simulink model "uas_main_latest"  (R2025a)
settings: Solver=FixedStepAuto  StartTime=0.0  StopTime=Inf  FixedStep=sample_time  RelTol=1e-3
model workspace: external: MAT-File (data not in the file)
values from neighbouring files (symbols this model uses):
  arm_length = 0.17    [test_uas_parameters.m]    (also in uas_parameters.m; uas_parameters_akin.m; uas_parameters_brushless.m = 0.046)
  drag_coefficient = 0.47    [uas_parameters.m]    (also in uas_parameters_akin.m; uas_parameters_brushless.m)
  g = 9.80665    [test_uas_parameters.m]    (also in uas_parameters.m; uas_parameters_akin.m; uas_parameters_brushless.m)
  inertia_xx = 0.007    [test_uas_parameters.m]    (also in uas_parameters.m; uas_parameters_akin.m; uas_parameters_brushless.m = 1.657171e-05)
  inertia_yy = 0.007    [test_uas_parameters.m]    (also in uas_parameters.m; uas_parameters_akin.m; uas_parameters_brushless.m = 1.6655602e-05)
  inertia_zz = 0.012    [test_uas_parameters.m]    (also in uas_parameters.m; uas_parameters_akin.m; uas_parameters_brushless.m = 2.9261652e-05)
  mass_drone = 0.68    [test_uas_parameters.m]    (also in uas_parameters.m; uas_parameters_akin.m; uas_parameters_brushless.m = 0.037)
  mass_total = mass_drone    (= 0.68)    [test_uas_parameters.m]    (also in uas_parameters.m; uas_parameters_akin.m; uas_parameters_brushless.m = 0.037)
  max_rot_velocity = 838    [uas_parameters.m]    (also in uas_parameters_akin.m; uas_parameters_brushless.m)
  mix_matrix = inv(motor_constant * allocation_matrix)    [test_uas_parameters.m]    (also in uas_parameters.m; uas_parameters_akin.m; uas_parameters_brushless.m)
  moment_constant = 0.016    [test_uas_parameters.m]    (also in uas_parameters.m; uas_parameters_akin.m; uas_parameters_brushless.m = 0.006)
  motor_constant = 8.54858e-06    [test_uas_parameters.m]    (also in uas_parameters.m; uas_parameters_akin.m; uas_parameters_brushless.m = 1.45e-08)
  publish_rate = sample_time    (= 0.04)    [test_uas_parameters.m]    (also in uas_parameters.m; uas_parameters_akin.m; uas_parameters_brushless.m)
  reference_area = pi * (75e-3)^2    (= 0.0176714586764)    [uas_parameters.m]    (also in uas_parameters_akin.m; uas_parameters_brushless.m)
  rotor_offset_top = 0.01    [uas_parameters.m]    (also in uas_parameters_akin.m; uas_parameters_brushless.m)
  route = route_scaled    [generate_route_for_simulink.m]    (also in uas_parameters.m = route_smooth; uas_parameters_akin.m = route_dense; uas_parameters_brushless.m = [0 0 1 ; 9 0 1 ; 9 9 1])
  sample_time = 4e-2    (= 0.04)    [test_uas_parameters.m]    (also in uas_parameters.m; uas_parameters_akin.m; uas_parameters_brushless.m)
  x0 = route_world(1,1)    [uas_parameters.m]    (also in uas_parameters_akin.m = route(1,1); uas_parameters_brushless.m = 36)
  y0 = route_world(1,2)    [uas_parameters.m]    (also in uas_parameters_akin.m = route(1,2); uas_parameters_brushless.m = 80)
  z0 = route_world(1,3)    [uas_parameters.m]    (also in uas_parameters_akin.m = route(1,3); uas_parameters_brushless.m = 1)
undefined symbols (not defined in the file or in its folder): Angular, Linear, poly_traj, Position, quat2rotm, X, Y, Z
libraries: nesl_utility x32, sm_lib x25, ros2lib x8, sim3dlib x1, uavsim3dlib x1, simulink x1, vrlib x1, simulink_extras x1
(part 2 of 2)

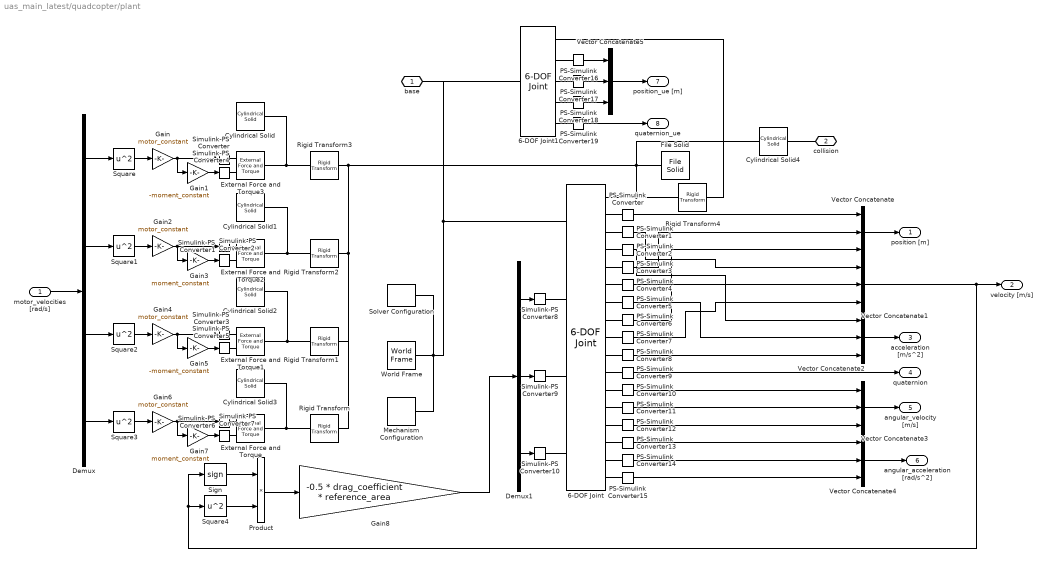
== system uas_main_latest/quadcopter/plant ==
  motor_velocities [rad/s] : Inport
  6-DOF Joint : sm_lib/Joints/6-DOF Joint  JointMode=Normal  CompositeWrenchDir=BaseOnFollower  CompositeWrenchFrame=BaseFrame  SenseConstraintForce=off  SenseConstraintTorque=off  SenseTotalForce=off  SenseTotalTorque=off  PxPositionTargetSpecify=on  PxPositionTargetPriority=High  PxPositionTargetValue=0  PxPositionTargetValueUnits=m  PxVelocityTargetSpecify=off  PxVelocityTargetPriority=High  PxVelocityTargetValue=0  PxVelocityTargetValueUnits=m/s  PxEquilibriumPosition=0  PxEquilibriumPositionUnits=m  PxSpringStiffness=0  PxSpringStiffnessUnits=N/m  PxDampingCoefficient=0  PxDampingCoefficientUnits=N/(m/s)  PxLowerLimitSpecify=off  PxLowerLimitBound=-1  PxLowerLimitBoundUnits=m  PxLowerLimitStiffness=1e6  PxLowerLimitStiffnessUnits=N/m  PxLowerLimitDamping=1e3  PxLowerLimitDampingUnits=N/(m/s)  PxLowerLimitTransitionRegionWidth=1e-4  PxLowerLimitTransitionRegionWidthUnits=m  PxUpperLimitSpecify=off  PxUpperLimitBound=1  PxUpperLimitBoundUnits=m  PxUpperLimitStiffness=1e6  PxUpperLimitStiffnessUnits=N/m  PxUpperLimitDamping=1e3  PxUpperLimitDampingUnits=N/(m/s)  PxUpperLimitTransitionRegionWidth=1e-4  PxUpperLimitTransitionRegionWidthUnits=m  PxTorqueActuationMode=InputTorque  PxMotionActuationMode=ComputedMotion  PxSensePosition=on  PxSenseVelocity=on  PxSenseAcceleration=on  PxSenseTorqueForce=off  PxSenseLowerLimitTorqueForce=off  PxSenseUpperLimitTorqueForce=off  PyPositionTargetSpecify=on  PyPositionTargetPriority=High  PyPositionTargetValue=0  PyPositionTargetValueUnits=m  PyVelocityTargetSpecify=off  PyVelocityTargetPriority=High  PyVelocityTargetValue=0  PyVelocityTargetValueUnits=m/s  PyEquilibriumPosition=0  PyEquilibriumPositionUnits=m  PySpringStiffness=0  PySpringStiffnessUnits=N/m  PyDampingCoefficient=0  PyDampingCoefficientUnits=N/(m/s)  PyLowerLimitSpecify=off  PyLowerLimitBound=-1  PyLowerLimitBoundUnits=m  PyLowerLimitStiffness=1e6  PyLowerLimitStiffnessUnits=N/m  PyLowerLimitDamping=1e3  PyLowerLimitDampingUnits=N/(m/s)  PyLowerLimitTransitionRegionWidth=1e-4  PyLowerLimitTransitionRegionWidthUnits=m  PyUpperLimitSpecify=off  PyUpperLimitBound=1  PyUpperLimitBoundUnits=m  PyUpperLimitStiffness=1e6  PyUpperLimitStiffnessUnits=N/m  PyUpperLimitDamping=1e3  PyUpperLimitDampingUnits=N/(m/s)  PyUpperLimitTransitionRegionWidth=1e-4  PyUpperLimitTransitionRegionWidthUnits=m  PyTorqueActuationMode=InputTorque  PyMotionActuationMode=ComputedMotion  PySensePosition=on  PySenseVelocity=on  PySenseAcceleration=on  PySenseTorqueForce=off  PySenseLowerLimitTorqueForce=off  PySenseUpperLimitTorqueForce=off  PzPositionTargetSpecify=on  PzPositionTargetPriority=High  PzPositionTargetValue=z0  PzPositionTargetValueUnits=m  PzVelocityTargetSpecify=off  PzVelocityTargetPriority=High  PzVelocityTargetValue=0  PzVelocityTargetValueUnits=m/s  PzEquilibriumPosition=0  PzEquilibriumPositionUnits=m  PzSpringStiffness=0  PzSpringStiffnessUnits=N/m  PzDampingCoefficient=0  PzDampingCoefficientUnits=N/(m/s)  PzLowerLimitSpecify=off  PzLowerLimitBound=-1  PzLowerLimitBoundUnits=m  PzLowerLimitStiffness=1e6  PzLowerLimitStiffnessUnits=N/m  PzLowerLimitDamping=1e3  PzLowerLimitDampingUnits=N/(m/s)  PzLowerLimitTransitionRegionWidth=1e-4  PzLowerLimitTransitionRegionWidthUnits=m  PzUpperLimitSpecify=off  PzUpperLimitBound=1  PzUpperLimitBoundUnits=m  PzUpperLimitStiffness=1e6  PzUpperLimitStiffnessUnits=N/m  PzUpperLimitDamping=1e3  PzUpperLimitDampingUnits=N/(m/s)  PzUpperLimitTransitionRegionWidth=1e-4  PzUpperLimitTransitionRegionWidthUnits=m  PzTorqueActuationMode=InputTorque  PzMotionActuationMode=ComputedMotion  PzSensePosition=on  PzSenseVelocity=on  PzSenseAcceleration=on  PzSenseTorqueForce=off  PzSenseLowerLimitTorqueForce=off  PzSenseUpperLimitTorqueForce=off  SphPositionTargetSpecify=on  SphPositionTargetPriority=High  SphPositionTargetRotationMethod=StandardAxis  SphPositionTargetFollAlignAxisA=+X  SphPositionTargetBaseAlignAxisA=+Y  SphPositionTargetFollAlignAxisB=+Y  SphPositionTargetBaseAlignAxisB=+Z  SphPositionTargetRotationStandardAxis=+Z  SphPositionTargetRotationAngle=0  SphPositionTargetRotationAngleUnits=deg  SphPositionTargetRotationArbitraryAxis=[0 0 1]  SphPositionTargetRotationSequenceAxes=FollowerAxes  SphPositionTargetRotationSequence=XYX  SphPositionTargetRotationSequenceAngles=[0 0 0]  SphPositionTargetRotationSequenceAnglesUnits=deg  SphPositionTargetRotationMatrix=[1 0 0; 0 1 0; 0 0 1]  SphPositionTargetQuaternion=[1 0 0 0]  SphVelocityTargetSpecify=off  SphVelocityTargetPriority=High  SphVelocityTargetValue=[0 0 0]  SphVelocityTargetValueUnits=deg/s  SphVelocityTargetInFollowerFrame=on  SphEqPosRotationMethod=None  SphEqPosFollAlignAxisA=+X  SphEqPosBaseAlignAxisA=+Y  SphEqPosFollAlignAxisB=+Y  SphEqPosBaseAlignAxisB=+Z  SphEqPosRotationStandardAxis=+Z  SphEqPosRotationAngle=0.0  SphEqPosRotationAngleUnits=deg  SphEqPosRotationArbitraryAxis=[0 0 1]  SphEqPosRotationSequenceAxes=FollowerAxes  SphEqPosRotationSequence=XYX  SphEqPosRotationSequenceAngles=[0 0 0]  SphEqPosRotationSequenceAnglesUnits=deg  SphEqPosRotationMatrix=[1 0 0; 0 1 0; 0 0 1]  SphEqPosQuaternion=[1 0 0 0]  SphSpringStiffness=0  SphSpringStiffnessUnits=N*m/deg  SphDampingCoefficient=0  SphDampingCoefficientUnits=N*m/(deg/s)  SphLowerLimitSpecify=off  SphLowerLimitBound=15  SphLowerLimitBoundUnits=deg  SphLowerLimitStiffness=1e4  SphLowerLimitStiffnessUnits=N*m/deg  SphLowerLimitDamping=10  SphLowerLimitDampingUnits=N*m/(deg/s)  SphLowerLimitTransitionRegionWidth=0.1  SphLowerLimitTransitionRegionWidthUnits=deg  SphUpperLimitSpecify=off  SphUpperLimitBound=45  SphUpperLimitBoundUnits=deg  SphUpperLimitStiffness=1e4  SphUpperLimitStiffnessUnits=N*m/deg  SphUpperLimitDamping=10  SphUpperLimitDampingUnits=N*m/(deg/s)  SphUpperLimitTransitionRegionWidth=0.1  SphUpperLimitTransitionRegionWidthUnits=deg  SphTorqueActuationMode=NoTorque  SphActuateTorqueX=off  SphActuateTorqueY=off  SphActuateTorqueZ=off  SphActuateTorque=off  SphActuationFrame=BaseFrame  SphSensePosition=on  SphSenseVelocityX=on  SphSenseVelocityY=on  SphSenseVelocityZ=on  SphSenseVelocity=off  SphSenseAccelerationX=on  SphSenseAccelerationY=on  SphSenseAccelerationZ=on  SphSenseAcceleration=off  SphSenseLowerLimitTorqueMag=off  SphSenseUpperLimitTorqueMag=off  SphSensingFrame=BaseFrame
  6-DOF Joint1 : sm_lib/Joints/6-DOF Joint  JointMode=Normal  CompositeWrenchDir=FollowerOnBase  CompositeWrenchFrame=BaseFrame  SenseConstraintForce=off  SenseConstraintTorque=off  SenseTotalForce=off  SenseTotalTorque=off  PxPositionTargetSpecify=off  PxPositionTargetPriority=High  PxPositionTargetValue=0  PxPositionTargetValueUnits=m  PxVelocityTargetSpecify=off  PxVelocityTargetPriority=High  PxVelocityTargetValue=0  PxVelocityTargetValueUnits=m/s  PxEquilibriumPosition=0  PxEquilibriumPositionUnits=m  PxSpringStiffness=0  PxSpringStiffnessUnits=N/m  PxDampingCoefficient=0  PxDampingCoefficientUnits=N/(m/s)  PxLowerLimitSpecify=off  PxLowerLimitBound=-1  PxLowerLimitBoundUnits=m  PxLowerLimitStiffness=1e6  PxLowerLimitStiffnessUnits=N/m  PxLowerLimitDamping=1e3  PxLowerLimitDampingUnits=N/(m/s)  PxLowerLimitTransitionRegionWidth=1e-4  PxLowerLimitTransitionRegionWidthUnits=m  PxUpperLimitSpecify=off  PxUpperLimitBound=1  PxUpperLimitBoundUnits=m  PxUpperLimitStiffness=1e6  PxUpperLimitStiffnessUnits=N/m  PxUpperLimitDamping=1e3  PxUpperLimitDampingUnits=N/(m/s)  PxUpperLimitTransitionRegionWidth=1e-4  PxUpperLimitTransitionRegionWidthUnits=m  PxTorqueActuationMode=NoTorque  PxMotionActuationMode=ComputedMotion  PxSensePosition=on  PxSenseVelocity=off  PxSenseAcceleration=off  PxSenseTorqueForce=off  PxSenseLowerLimitTorqueForce=off  PxSenseUpperLimitTorqueForce=off  PyPositionTargetSpecify=off  PyPositionTargetPriority=High  PyPositionTargetValue=0  PyPositionTargetValueUnits=m  PyVelocityTargetSpecify=off  PyVelocityTargetPriority=High  PyVelocityTargetValue=0  PyVelocityTargetValueUnits=m/s  PyEquilibriumPosition=0  PyEquilibriumPositionUnits=m  PySpringStiffness=0  PySpringStiffnessUnits=N/m  PyDampingCoefficient=0  PyDampingCoefficientUnits=N/(m/s)  PyLowerLimitSpecify=off  PyLowerLimitBound=-1  PyLowerLimitBoundUnits=m  PyLowerLimitStiffness=1e6  PyLowerLimitStiffnessUnits=N/m  PyLowerLimitDamping=1e3  PyLowerLimitDampingUnits=N/(m/s)  PyLowerLimitTransitionRegionWidth=1e-4  PyLowerLimitTransitionRegionWidthUnits=m  PyUpperLimitSpecify=off  PyUpperLimitBound=1  PyUpperLimitBoundUnits=m  PyUpperLimitStiffness=1e6  PyUpperLimitStiffnessUnits=N/m  PyUpperLimitDamping=1e3  PyUpperLimitDampingUnits=N/(m/s)  PyUpperLimitTransitionRegionWidth=1e-4  PyUpperLimitTransitionRegionWidthUnits=m  PyTorqueActuationMode=NoTorque  PyMotionActuationMode=ComputedMotion  PySensePosition=on  PySenseVelocity=off  PySenseAcceleration=off  PySenseTorqueForce=off  PySenseLowerLimitTorqueForce=off  PySenseUpperLimitTorqueForce=off  PzPositionTargetSpecify=off  PzPositionTargetPriority=High  PzPositionTargetValue=0  PzPositionTargetValueUnits=m  PzVelocityTargetSpecify=off  PzVelocityTargetPriority=High  PzVelocityTargetValue=0  PzVelocityTargetValueUnits=m/s  PzEquilibriumPosition=0  PzEquilibriumPositionUnits=m  PzSpringStiffness=0  PzSpringStiffnessUnits=N/m  PzDampingCoefficient=0  PzDampingCoefficientUnits=N/(m/s)  PzLowerLimitSpecify=off  PzLowerLimitBound=-1  PzLowerLimitBoundUnits=m  PzLowerLimitStiffness=1e6  PzLowerLimitStiffnessUnits=N/m  PzLowerLimitDamping=1e3  PzLowerLimitDampingUnits=N/(m/s)  PzLowerLimitTransitionRegionWidth=1e-4  PzLowerLimitTransitionRegionWidthUnits=m  PzUpperLimitSpecify=off  PzUpperLimitBound=1  PzUpperLimitBoundUnits=m  PzUpperLimitStiffness=1e6  PzUpperLimitStiffnessUnits=N/m  PzUpperLimitDamping=1e3  PzUpperLimitDampingUnits=N/(m/s)  PzUpperLimitTransitionRegionWidth=1e-4  PzUpperLimitTransitionRegionWidthUnits=m  PzTorqueActuationMode=NoTorque  PzMotionActuationMode=ComputedMotion  PzSensePosition=on  PzSenseVelocity=off  PzSenseAcceleration=off  PzSenseTorqueForce=off  PzSenseLowerLimitTorqueForce=off  PzSenseUpperLimitTorqueForce=off  SphPositionTargetSpecify=off  SphPositionTargetPriority=High  SphPositionTargetRotationMethod=None  SphPositionTargetFollAlignAxisA=+X  SphPositionTargetBaseAlignAxisA=+Y  SphPositionTargetFollAlignAxisB=+Y  SphPositionTargetBaseAlignAxisB=+Z  SphPositionTargetRotationStandardAxis=+Z  SphPositionTargetRotationAngle=0.0  SphPositionTargetRotationAngleUnits=deg  SphPositionTargetRotationArbitraryAxis=[0 0 1]  SphPositionTargetRotationSequenceAxes=FollowerAxes  SphPositionTargetRotationSequence=XYX  SphPositionTargetRotationSequenceAngles=[0 0 0]  SphPositionTargetRotationSequenceAnglesUnits=deg  SphPositionTargetRotationMatrix=[1 0 0; 0 1 0; 0 0 1]  SphPositionTargetQuaternion=[1 0 0 0]  SphVelocityTargetSpecify=off  SphVelocityTargetPriority=High  SphVelocityTargetValue=[0 0 0]  SphVelocityTargetValueUnits=deg/s  SphVelocityTargetInFollowerFrame=on  SphEqPosRotationMethod=None  SphEqPosFollAlignAxisA=+X  SphEqPosBaseAlignAxisA=+Y  SphEqPosFollAlignAxisB=+Y  SphEqPosBaseAlignAxisB=+Z  SphEqPosRotationStandardAxis=+Z  SphEqPosRotationAngle=0.0  SphEqPosRotationAngleUnits=deg  SphEqPosRotationArbitraryAxis=[0 0 1]  SphEqPosRotationSequenceAxes=FollowerAxes  SphEqPosRotationSequence=XYX  SphEqPosRotationSequenceAngles=[0 0 0]  SphEqPosRotationSequenceAnglesUnits=deg  SphEqPosRotationMatrix=[1 0 0; 0 1 0; 0 0 1]  SphEqPosQuaternion=[1 0 0 0]  SphSpringStiffness=0  SphSpringStiffnessUnits=N*m/deg  SphDampingCoefficient=0  SphDampingCoefficientUnits=N*m/(deg/s)  SphLowerLimitSpecify=off  SphLowerLimitBound=15  SphLowerLimitBoundUnits=deg  SphLowerLimitStiffness=1e4  SphLowerLimitStiffnessUnits=N*m/deg  SphLowerLimitDamping=10  SphLowerLimitDampingUnits=N*m/(deg/s)  SphLowerLimitTransitionRegionWidth=0.1  SphLowerLimitTransitionRegionWidthUnits=deg  SphUpperLimitSpecify=off  SphUpperLimitBound=45  SphUpperLimitBoundUnits=deg  SphUpperLimitStiffness=1e4  SphUpperLimitStiffnessUnits=N*m/deg  SphUpperLimitDamping=10  SphUpperLimitDampingUnits=N*m/(deg/s)  SphUpperLimitTransitionRegionWidth=0.1  SphUpperLimitTransitionRegionWidthUnits=deg  SphTorqueActuationMode=NoTorque  SphActuateTorqueX=off  SphActuateTorqueY=off  SphActuateTorqueZ=off  SphActuateTorque=off  SphActuationFrame=BaseFrame  SphSensePosition=on  SphSenseVelocityX=off  SphSenseVelocityY=off  SphSenseVelocityZ=off  SphSenseVelocity=off  SphSenseAccelerationX=off  SphSenseAccelerationY=off  SphSenseAccelerationZ=off  SphSenseAcceleration=off  SphSenseLowerLimitTorqueMag=off  SphSenseUpperLimitTorqueMag=off  SphSensingFrame=BaseFrame
  Cylindrical Solid : sm_lib/Body Elements/Cylindrical Solid  CylinderRadius=100  CylinderRadiusUnits=mm  CylinderLength=1  CylinderLengthUnits=mm  ExportEntireGeometry=off  InertiaType=CalculateFromGeometry  BasedOnType=Density  Density=0  DensityUnits=kg/m^3  Mass=1  MassUnits=kg  CenterOfMass=[0 0 0]  CenterOfMassUnits=m  MomentsOfInertia=[1 1 1]  MomentsOfInertiaUnits=kg*m^2  ProductsOfInertia=[0 0 0]  ProductsOfInertiaUnits=kg*m^2  GraphicType=FromGeometry  MarkerShape=Sphere  MarkerSize=10  GraphicVisPropType=SimpleVisualProperties  GraphicDiffuseColor=[1.0 0.0 0.0]  GraphicOpacity=0.5  GraphicSpecularColor=[0.5 0.5 0.5 1.0]  GraphicAmbientColor=[0.15 0.15 0.15 1.0]  GraphicEmissiveColor=[0.0 0.0 0.0 1.0]  GraphicShininess=75  DoExposeReferenceFrame=on  SerializedFrames=<Frames/>
  Cylindrical Solid1 : sm_lib/Body Elements/Cylindrical Solid  CylinderRadius=100  CylinderRadiusUnits=mm  CylinderLength=1  CylinderLengthUnits=mm  ExportEntireGeometry=off  InertiaType=CalculateFromGeometry  BasedOnType=Density  Density=0  DensityUnits=kg/m^3  Mass=1  MassUnits=kg  CenterOfMass=[0 0 0]  CenterOfMassUnits=m  MomentsOfInertia=[1 1 1]  MomentsOfInertiaUnits=kg*m^2  ProductsOfInertia=[0 0 0]  ProductsOfInertiaUnits=kg*m^2  GraphicType=FromGeometry  MarkerShape=Sphere  MarkerSize=10  GraphicVisPropType=SimpleVisualProperties  GraphicDiffuseColor=[0 1 0]  GraphicOpacity=0.5  GraphicSpecularColor=[0.5 0.5 0.5 1.0]  GraphicAmbientColor=[0.15 0.15 0.15 1.0]  GraphicEmissiveColor=[0.0 0.0 0.0 1.0]  GraphicShininess=75  DoExposeReferenceFrame=on  SerializedFrames=<Frames/>
  Cylindrical Solid2 : sm_lib/Body Elements/Cylindrical Solid  CylinderRadius=100  CylinderRadiusUnits=mm  CylinderLength=1  CylinderLengthUnits=mm  ExportEntireGeometry=off  InertiaType=CalculateFromGeometry  BasedOnType=Density  Density=0  DensityUnits=kg/m^3  Mass=1  MassUnits=kg  CenterOfMass=[0 0 0]  CenterOfMassUnits=m  MomentsOfInertia=[1 1 1]  MomentsOfInertiaUnits=kg*m^2  ProductsOfInertia=[0 0 0]  ProductsOfInertiaUnits=kg*m^2  GraphicType=FromGeometry  MarkerShape=Sphere  MarkerSize=10  GraphicVisPropType=SimpleVisualProperties  GraphicDiffuseColor=[0 0 1]  GraphicOpacity=0.5  GraphicSpecularColor=[0.5 0.5 0.5 1.0]  GraphicAmbientColor=[0.15 0.15 0.15 1.0]  GraphicEmissiveColor=[0.0 0.0 0.0 1.0]  GraphicShininess=75  DoExposeReferenceFrame=on  SerializedFrames=<Frames/>
  Cylindrical Solid3 : sm_lib/Body Elements/Cylindrical Solid  CylinderRadius=100  CylinderRadiusUnits=mm  CylinderLength=1  CylinderLengthUnits=mm  ExportEntireGeometry=off  InertiaType=CalculateFromGeometry  BasedOnType=Density  Density=0  DensityUnits=kg/m^3  Mass=1  MassUnits=kg  CenterOfMass=[0 0 0]  CenterOfMassUnits=m  MomentsOfInertia=[1 1 1]  MomentsOfInertiaUnits=kg*m^2  ProductsOfInertia=[0 0 0]  ProductsOfInertiaUnits=kg*m^2  GraphicType=FromGeometry  MarkerShape=Sphere  MarkerSize=10  GraphicVisPropType=SimpleVisualProperties  GraphicDiffuseColor=[0 0 1]  GraphicOpacity=0.5  GraphicSpecularColor=[0.5 0.5 0.5 1.0]  GraphicAmbientColor=[0.15 0.15 0.15 1.0]  GraphicEmissiveColor=[0.0 0.0 0.0 1.0]  GraphicShininess=75  DoExposeReferenceFrame=on  SerializedFrames=<Frames/>
  Cylindrical Solid4 : sm_lib/Body Elements/Cylindrical Solid  CylinderRadius=0.27  CylinderRadiusUnits=m  CylinderLength=0.3  CylinderLengthUnits=m  ExportEntireGeometry=on  InertiaType=CalculateFromGeometry  BasedOnType=Density  Density=0  DensityUnits=kg/m^3  Mass=1  MassUnits=kg  CenterOfMass=[0 0 0]  CenterOfMassUnits=m  MomentsOfInertia=[1 1 1]  MomentsOfInertiaUnits=kg*m^2  ProductsOfInertia=[0 0 0]  ProductsOfInertiaUnits=kg*m^2  GraphicType=FromGeometry  MarkerShape=Sphere  MarkerSize=10  GraphicVisPropType=SimpleVisualProperties  GraphicDiffuseColor=[0.5 0.5 0.5]  GraphicOpacity=0.2  GraphicSpecularColor=[0.5 0.5 0.5 1.0]  GraphicAmbientColor=[0.15 0.15 0.15 1.0]  GraphicEmissiveColor=[0.0 0.0 0.0 1.0]  GraphicShininess=75  DoExposeReferenceFrame=on  SerializedFrames=<Frames/>
  Demux : Demux
  Demux1 : Demux  Outputs=3
  External Force and Torque{,1..3} (4 alike) : sm_lib/Forces and Torques/External Force and Torque  EnableForceX=off  EnableForceY=off  EnableForceZ=on  EnableForce=off  ForceResolutionFrame=AttachedFrame  EnableTorqueX=off  EnableTorqueY=off  EnableTorqueZ=on  EnableTorque=off  TorqueResolutionFrame=AttachedFrame
  File Solid : sm_lib/Body Elements/File Solid  ExtGeomFileName=uas_geometry.stl  UnitType=Custom  ExtGeomFileUnits=m  StepReaderType=HEX  ExportConvexHullGeometry=off  InertiaType=Custom  BasedOnType=DensityFromFile  Density=1000  DensityUnits=kg/m^3  Mass=mass_drone  MassUnits=kg  CenterOfMass=[0 0 0]  CenterOfMassUnits=m  MomentsOfInertia=[inertia_xx inertia_yy inertia_zz]  MomentsOfInertiaUnits=kg*m^2  ProductsOfInertia=[0 0 0]  ProductsOfInertiaUnits=kg*m^2  GraphicType=FromGeometry  MarkerShape=Sphere  MarkerSize=10  GraphicVisPropType=SimpleVisualProperties  GraphicDiffuseColor=[1.0 1.0 1.0]  GraphicOpacity=1.0  GraphicSpecularColor=[0.5 0.5 0.5 1.0]  GraphicAmbientColor=[0.15 0.15 0.15 1.0]  GraphicEmissiveColor=[0.0 0.0 0.0 1.0]  GraphicShininess=75  DoExposeReferenceFrame=on  SerializedFrames=<Frames/>
  Gain{,2,4,6} (4 alike) : Gain  Gain=motor_constant
  Gain1 : Gain  Gain=-moment_constant
  Gain3 : Gain  Gain=moment_constant
  Gain5 : Gain  Gain=-moment_constant
  Gain7 : Gain  Gain=moment_constant
  Gain8 : Gain  Gain=-0.5 * drag_coefficient * reference_area
  Mechanism Configuration : sm_lib/Utilities/Mechanism Configuration  UniformGravity=Constant  GravityVector=[0 0 -9.80665]  GravityVectorUnits=m/s^2  LinearizationDelta=0.001  JointModeTransitionNonlinearIterations=2
  PS-Simulink Converter{,1..19} (20 alike) : nesl_utility/PS-Simulink Converter  PhysicalDomain=network_engine_domain  SubClassName=ps_output  LeftPortType=input  RightPortType=output  PseudoPeriodic=off  Frequencies=[]  VectorFormat=1-D array  Unit=inherit  AffineConversion=off
  Product : Product
  Rigid Transform : sm_lib/Frames and Transforms/Rigid Transform  RotationMethod=None  FollAlignAxisA=+X  BaseAlignAxisA=+Y  FollAlignAxisB=+Y  BaseAlignAxisB=+Z  RotationStandardAxis=+Z  RotationAngle=0.0  RotationAngleUnits=deg  RotationArbitraryAxis=[0 0 1]  RotationSequenceAxes=FollowerAxes  RotationSequence=XYX  RotationSequenceAngles=[0 0 0]  RotationSequenceAnglesUnits=deg  RotationMatrix=[1 0 0; 0 1 0; 0 0 1]  Quaternion=[1 0 0 0]  TranslationMethod=Cartesian  TranslationCartesianOffset=[0 -arm_length rotor_offset_top]  TranslationCartesianOffsetUnits=m  TranslationStandardAxis=+Z  TranslationStandardOffset=0  TranslationStandardOffsetUnits=m  TranslationROffset=0  TranslationROffsetUnits=m  TranslationThetaOffset=0  TranslationThetaOffsetUnits=deg  TranslationZOffset=0  TranslationZOffsetUnits=m
  Rigid Transform1 : sm_lib/Frames and Transforms/Rigid Transform  RotationMethod=None  FollAlignAxisA=+X  BaseAlignAxisA=+Y  FollAlignAxisB=+Y  BaseAlignAxisB=+Z  RotationStandardAxis=+Z  RotationAngle=0.0  RotationAngleUnits=deg  RotationArbitraryAxis=[0 0 1]  RotationSequenceAxes=FollowerAxes  RotationSequence=XYX  RotationSequenceAngles=[0 0 0]  RotationSequenceAnglesUnits=deg  RotationMatrix=[1 0 0; 0 1 0; 0 0 1]  Quaternion=[1 0 0 0]  TranslationMethod=Cartesian  TranslationCartesianOffset=[-arm_length 0 rotor_offset_top]  TranslationCartesianOffsetUnits=m  TranslationStandardAxis=+Z  TranslationStandardOffset=0  TranslationStandardOffsetUnits=m  TranslationROffset=0  TranslationROffsetUnits=m  TranslationThetaOffset=0  TranslationThetaOffsetUnits=deg  TranslationZOffset=0  TranslationZOffsetUnits=m
  Rigid Transform2 : sm_lib/Frames and Transforms/Rigid Transform  RotationMethod=None  FollAlignAxisA=+X  BaseAlignAxisA=+Y  FollAlignAxisB=+Y  BaseAlignAxisB=+Z  RotationStandardAxis=+Z  RotationAngle=0.0  RotationAngleUnits=deg  RotationArbitraryAxis=[0 0 1]  RotationSequenceAxes=FollowerAxes  RotationSequence=XYX  RotationSequenceAngles=[0 0 0]  RotationSequenceAnglesUnits=deg  RotationMatrix=[1 0 0; 0 1 0; 0 0 1]  Quaternion=[1 0 0 0]  TranslationMethod=Cartesian  TranslationCartesianOffset=[0 arm_length rotor_offset_top]  TranslationCartesianOffsetUnits=m  TranslationStandardAxis=+Z  TranslationStandardOffset=0  TranslationStandardOffsetUnits=m  TranslationROffset=0  TranslationROffsetUnits=m  TranslationThetaOffset=0  TranslationThetaOffsetUnits=deg  TranslationZOffset=0  TranslationZOffsetUnits=m
  Rigid Transform3 : sm_lib/Frames and Transforms/Rigid Transform  RotationMethod=None  FollAlignAxisA=+X  BaseAlignAxisA=+Y  FollAlignAxisB=+Y  BaseAlignAxisB=+Z  RotationStandardAxis=+Z  RotationAngle=0.0  RotationAngleUnits=deg  RotationArbitraryAxis=[0 0 1]  RotationSequenceAxes=FollowerAxes  RotationSequence=XYX  RotationSequenceAngles=[0 0 0]  RotationSequenceAnglesUnits=deg  RotationMatrix=[1 0 0; 0 1 0; 0 0 1]  Quaternion=[1 0 0 0]  TranslationMethod=Cartesian  TranslationCartesianOffset=[arm_length 0 rotor_offset_top]  TranslationCartesianOffsetUnits=m  TranslationStandardAxis=+Z  TranslationStandardOffset=0  TranslationStandardOffsetUnits=m  TranslationROffset=0  TranslationROffsetUnits=m  TranslationThetaOffset=0  TranslationThetaOffsetUnits=deg  TranslationZOffset=0  TranslationZOffsetUnits=m
  Rigid Transform4 : sm_lib/Frames and Transforms/Rigid Transform  RotationMethod=None  FollAlignAxisA=+X  BaseAlignAxisA=+Y  FollAlignAxisB=+Y  BaseAlignAxisB=+Z  RotationStandardAxis=+Z  RotationAngle=0.0  RotationAngleUnits=deg  RotationArbitraryAxis=[0 0 1]  RotationSequenceAxes=FollowerAxes  RotationSequence=XYX  RotationSequenceAngles=[0 0 0]  RotationSequenceAnglesUnits=deg  RotationMatrix=[1 0 0; 0 1 0; 0 0 1]  Quaternion=[1 0 0 0]  TranslationMethod=StandardAxis  TranslationCartesianOffset=[0 0 0]  TranslationCartesianOffsetUnits=m  TranslationStandardAxis=-Z  TranslationStandardOffset=0.15  TranslationStandardOffsetUnits=m  TranslationROffset=0  TranslationROffsetUnits=m  TranslationThetaOffset=0  TranslationThetaOffsetUnits=deg  TranslationZOffset=0  TranslationZOffsetUnits=m
  Sign : Signum
  Simulink-PS Converter{,1..10} (11 alike) : nesl_utility/Simulink-PS Converter  PhysicalDomain=network_engine_domain  SubClassName=ps_input  LeftPortType=input  RightPortType=output  PseudoPeriodic=off  Frequencies=[]  NoiseDistribution=none  NoiseParameters=[]  Unit=1  AffineConversion=off  FilteringAndDerivatives=provide  SimscapeFilterOrder=1  InputFilterTimeConstant=0.001  UdotUserProvided=0
  Solver Configuration : nesl_utility/Solver Configuration  PhysicalDomain=network_engine_domain  SubClassName=solver  LeftPortType=input  RightPortType=generic  Tones=[]  Harmonics=[]  SimulateNoise=off  Profile=off  UseLocalSampling=off  EnableSwitchedLinearOptims=on  FrequencyDomain=off  UseCCode=off  RelTol=0.001  AbsTol=1e-06  MinStep=1e-09  ToWorkspace=off  RevertToSquareIcSolve=off  NumHomotopyIterations=100  PhasorMode=off  PhasorModeNumHarmonics=1  ConsistencySolver=NEWTON_FTOL  IndexReductionMethod=DerivativeReplacement  DoDC=off  ResidualTolerance=1e-09  ConsistencyTolSource=GLOBAL  ConsistencyAbsTol=0.001  ConsistencyRelTol=0.001  ConsistencyTolFactor=0.001  UseLocalSolver=off  LocalSolverChoice=NE_BACKWARD_EULER_ADVANCER  ResolveIndetEquations=on  FunctionEvalNumThread=1  LocalSolverSampleTime=0.001  DoFixedCost=off  MaxNonlinIter=3  MaxModeIter=2  ComputeImpulses=off  ImpulseIterations=2  LinearAlgebra=Sparse  LinearAlgebraNumThread=0  EquationFormulation=NE_TIME_EF  DelaysMemoryBudget=1024  AutomaticFiltering=on  FilteringTimeConstant=0.001  PartitionStorageMethod=AS_NEEDED  PartitionMemoryBudget=1024  PartitionMethod=FAST  MultibodyUseLocalSolver=off  MultibodyLocalSolverChoice=ODE1  MultibodyLocalSolverSampleTime=0.001
  Square{,1..4} (5 alike) : Math  Operator=square
  Vector Concatenate{,1..5} (6 alike) : Concatenate  NumInputs=3  Mode=Multidimensional array
  World Frame : sm_lib/Frames and Transforms/World Frame
  base : PMIOPort  Side=Right
  collision : PMIOPort  Port=2  Side=Right
  position [m] : Outport
  velocity [m/s] : Outport  Port=2
  acceleration [m/s^2] : Outport  Port=3
  quaternion : Outport  Port=4  PortDimensions=[1 4]
  angular_velocity [m/s] : Outport  Port=5
  angular_acceleration [rad/s^2] : Outport  Port=6
  position_ue [m] : Outport  Port=7
  quaternion_ue : Outport  Port=8
  wires:
  Square/1 -> Gain/1
  Gain/1 -> Gain1/1, Simulink-PS Converter/1
  Gain1/1 -> Simulink-PS Converter4/1
  Square1/1 -> Gain2/1
  Gain2/1 -> Gain3/1, Simulink-PS Converter1/1
  Gain3/1 -> Simulink-PS Converter2/1
  Gain5/1 -> Simulink-PS Converter5/1
  Square2/1 -> Gain4/1
  Gain4/1 -> Gain5/1, Simulink-PS Converter3/1
  Gain7/1 -> Simulink-PS Converter7/1
  Square3/1 -> Gain6/1
  Gain6/1 -> Gain7/1, Simulink-PS Converter6/1
  Demux/1 -> Square/1
  Demux/2 -> Square1/1
  Demux/3 -> Square2/1
  Demux/4 -> Square3/1
  motor_velocities [rad/s]/1 -> Demux/1
  Vector Concatenate/1 -> position [m]/1
  Vector Concatenate1/1 -> velocity [m/s]/1, Sign/1, Square4/1
  Vector Concatenate2/1 -> acceleration [m/s^2]/1
  PS-Simulink Converter9/1 -> quaternion/1
  Vector Concatenate3/1 -> angular_velocity [m/s]/1
  Vector Concatenate4/1 -> angular_acceleration [rad/s^2]/1
  PS-Simulink Converter/1 -> Vector Concatenate/1
  PS-Simulink Converter3/1 -> Vector Concatenate/2
  PS-Simulink Converter6/1 -> Vector Concatenate/3
  PS-Simulink Converter1/1 -> Vector Concatenate1/1
  PS-Simulink Converter4/1 -> Vector Concatenate1/2
  PS-Simulink Converter7/1 -> Vector Concatenate1/3
  PS-Simulink Converter2/1 -> Vector Concatenate2/1
  PS-Simulink Converter5/1 -> Vector Concatenate2/2
  PS-Simulink Converter8/1 -> Vector Concatenate2/3
  PS-Simulink Converter10/1 -> Vector Concatenate3/1
  PS-Simulink Converter11/1 -> Vector Concatenate3/2
  PS-Simulink Converter12/1 -> Vector Concatenate3/3
  PS-Simulink Converter13/1 -> Vector Concatenate4/1
  PS-Simulink Converter14/1 -> Vector Concatenate4/2
  PS-Simulink Converter15/1 -> Vector Concatenate4/3
  Demux1/1 -> Simulink-PS Converter8/1
  Demux1/2 -> Simulink-PS Converter9/1
  Demux1/3 -> Simulink-PS Converter10/1
  Gain8/1 -> Demux1/1
  Vector Concatenate5/1 -> position_ue [m]/1
  PS-Simulink Converter16/1 -> Vector Concatenate5/1
  PS-Simulink Converter17/1 -> Vector Concatenate5/2
  PS-Simulink Converter18/1 -> Vector Concatenate5/3
  PS-Simulink Converter19/1 -> quaternion_ue/1
  Product/1 -> Gain8/1
  Sign/1 -> Product/1
  Square4/1 -> Product/2
  connections:
  Rigid Transform/LConn1 -- Rigid Transform1/LConn1 -- Rigid Transform2/LConn1 -- Rigid Transform3/LConn1 -- Cylindrical Solid4/RConn1 -- File Solid/RConn1 -- Rigid Transform4/LConn1 -- 6-DOF Joint/RConn1
  World Frame/RConn1 -- 6-DOF Joint1/LConn1 -- base/RConn1 -- 6-DOF Joint/LConn1 -- Mechanism Configuration/RConn1 -- Solver Configuration/RConn1
  External Force and Torque3/RConn1 -- Cylindrical Solid/RConn1 -- Rigid Transform3/RConn1
  External Force and Torque2/RConn1 -- Cylindrical Solid1/RConn1 -- Rigid Transform2/RConn1
  External Force and Torque1/RConn1 -- Cylindrical Solid2/RConn1 -- Rigid Transform1/RConn1
  External Force and Torque/RConn1 -- Cylindrical Solid3/RConn1 -- Rigid Transform/RConn1
  Simulink-PS Converter/RConn1 -- External Force and Torque3/LConn1
  Simulink-PS Converter4/RConn1 -- External Force and Torque3/LConn2
  Simulink-PS Converter1/RConn1 -- External Force and Torque2/LConn1
  Simulink-PS Converter2/RConn1 -- External Force and Torque2/LConn2
  Simulink-PS Converter3/RConn1 -- External Force and Torque1/LConn1
  Simulink-PS Converter5/RConn1 -- External Force and Torque1/LConn2
  Simulink-PS Converter6/RConn1 -- External Force and Torque/LConn1
  Simulink-PS Converter7/RConn1 -- External Force and Torque/LConn2
  PS-Simulink Converter/LConn1 -- 6-DOF Joint/RConn2
  6-DOF Joint/RConn3 -- PS-Simulink Converter1/LConn1
  6-DOF Joint/RConn4 -- PS-Simulink Converter2/LConn1
  6-DOF Joint/RConn5 -- PS-Simulink Converter3/LConn1
  PS-Simulink Converter4/LConn1 -- 6-DOF Joint/RConn6
  PS-Simulink Converter5/LConn1 -- 6-DOF Joint/RConn7
  PS-Simulink Converter6/LConn1 -- 6-DOF Joint/RConn8
  PS-Simulink Converter7/LConn1 -- 6-DOF Joint/RConn9
  6-DOF Joint/RConn11 -- PS-Simulink Converter9/LConn1
  6-DOF Joint/RConn10 -- PS-Simulink Converter8/LConn1
  6-DOF Joint/RConn17 -- PS-Simulink Converter15/LConn1
  6-DOF Joint/RConn16 -- PS-Simulink Converter14/LConn1
  6-DOF Joint/RConn15 -- PS-Simulink Converter13/LConn1
  6-DOF Joint/RConn14 -- PS-Simulink Converter12/LConn1
  6-DOF Joint/RConn13 -- PS-Simulink Converter11/LConn1
  6-DOF Joint/RConn12 -- PS-Simulink Converter10/LConn1
  Simulink-PS Converter8/RConn1 -- 6-DOF Joint/LConn2
  Simulink-PS Converter10/RConn1 -- 6-DOF Joint/LConn4
  Simulink-PS Converter9/RConn1 -- 6-DOF Joint/LConn3
  PS-Simulink Converter16/LConn1 -- 6-DOF Joint1/RConn2
  PS-Simulink Converter17/LConn1 -- 6-DOF Joint1/RConn3
  PS-Simulink Converter18/LConn1 -- 6-DOF Joint1/RConn4
  PS-Simulink Converter19/LConn1 -- 6-DOF Joint1/RConn5
  6-DOF Joint1/RConn1 -- Rigid Transform4/RConn1
  collision/RConn1 -- Cylindrical Solid4/LConn1

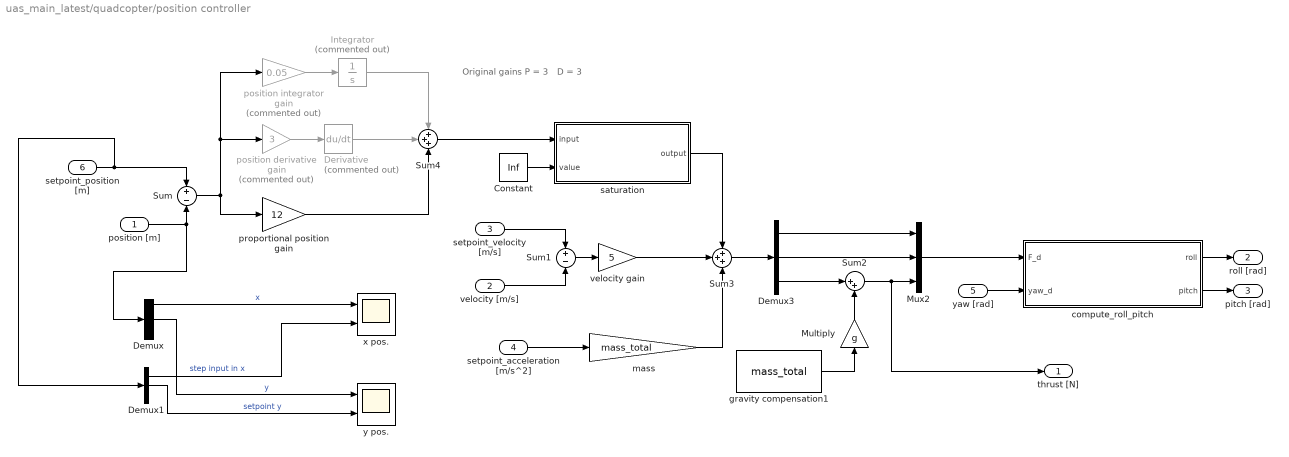
== system uas_main_latest/quadcopter/position controller ==
  note: D = 3
  note: Original gains P = 3
  position [m] : Inport
  velocity [m/s] : Inport  Port=2
  setpoint_velocity [m/s] : Inport  Port=3
  setpoint_acceleration [m/s^2] : Inport  Port=4
  yaw [rad] : Inport  Port=5
  setpoint_position [m] : Inport  Port=6
  Constant : Constant  Value=Inf
  Demux : Demux  Outputs=3
  Demux1 : Demux  Outputs=3
  Demux3 : Demux  Outputs=3
  Derivative : Derivative  Commented=on
  Integrator : Integrator  Commented=on
  Multiply : Gain  Gain=g
  Mux2 : Mux  Inputs=3
  Sum : Sum  Inputs=+|-
  Sum1 : Sum  Inputs=+|-
  Sum2 : Sum  Inputs=|++
  Sum3 : Sum  Inputs=+++
  Sum4 : Sum  Inputs=+++
  compute_roll_pitch : MATLAB Function  TreatAsAtomicUnit=on
  gravity compensation1 : Constant  Value=mass_total  VectorParams1D=off
  mass : Gain  Gain=mass_total
  position derivative gain : Gain  Commented=on  Gain=3
  position integrator gain : Gain  Commented=on  Gain=0.05
  proportional position gain : Gain  Gain=12
  saturation : Subsystem
  velocity gain : Gain  Gain=5
  x pos. : Scope  NumInputPorts=2
      settings: ActiveDisplayYMinimum=-0.16066462489966371  ActiveDisplayYMaximum=8.3113664097172286  DataLoggingVariableName=ScopeData8
  y pos. : Scope  NumInputPorts=2
      settings: ActiveDisplayYMinimum=-0.89466828166511936  ActiveDisplayYMaximum=7.1827417817229824  DataLoggingVariableName=ScopeData10
  thrust [N] : Outport
  roll [rad] : Outport  Port=2
  pitch [rad] : Outport  Port=3
  wires:
  saturation/1(output) -> Sum3/1
  gravity compensation1/1 -> Multiply/1
  velocity [m/s]/1 -> Sum1/2
  Demux3/3 -> Sum2/1
  mass/1 -> Sum3/3
  Constant/1 -> saturation/2(value)
  Sum2/1 -> thrust [N]/1, Mux2/3
  Sum1/1 -> velocity gain/1
  velocity gain/1 -> Sum3/2
  Sum3/1 -> Demux3/1
  Demux3/1 -> Mux2/1
  Mux2/1 -> compute_roll_pitch/1(F_d)
  Demux3/2 -> Mux2/2
  compute_roll_pitch/1(roll) -> roll [rad]/1
  Multiply/1 -> Sum2/2
  setpoint_position [m]/1 -> Demux1/1, Sum/1
  compute_roll_pitch/2(pitch) -> pitch [rad]/1
  position [m]/1 -> Demux/1, Sum/2
  yaw [rad]/1 -> compute_roll_pitch/2(yaw_d)
  setpoint_velocity [m/s]/1 -> Sum1/1
  setpoint_acceleration [m/s^2]/1 -> mass/1
  Sum/1 -> proportional position gain/1, position derivative gain/1, position integrator gain/1
  position derivative gain/1 -> Derivative/1
  Derivative/1 -> Sum4/2
  proportional position gain/1 -> Sum4/3
  Integrator/1 -> Sum4/1
  position integrator gain/1 -> Integrator/1
  Sum4/1 -> saturation/1(input)
  Demux/1 -> x pos./1  "x"
  Demux1/1 -> x pos./2  "step input in x"
  Demux/2 -> y pos./1  "y"
  Demux1/2 -> y pos./2  "setpoint y"

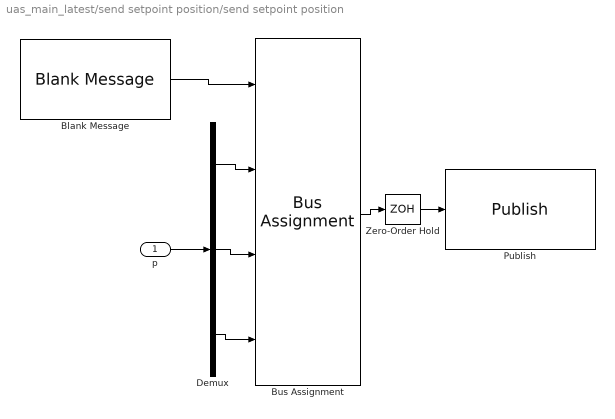
== system uas_main_latest/send setpoint position/send setpoint position ==
  p : Inport
  Blank Message : ros2lib/Blank Message  messageClass=Message  entityType=crazyflie_interfaces/Position  messageType=crazyflie_interfaces/Position  SampleTime=inf
  Bus Assignment : BusAssignment  AssignedSignals=Position.X,Position.Y,Position.Z
  Demux : Demux  Outputs=3
  Publish : ros2lib/Publish  topicSource=Specify your own  topic=/cf231/cmd_position  messageType=crazyflie_interfaces/Position  QOSHistory=Keep last  QOSDepth=1  QOSReliability=Reliable  QOSDurability=Volatile  QOSDeadline=Inf  QOSLifespan=Inf  QOSLiveliness=Automatic  QOSLeaseDuration=Inf  QOSAvoidROSNamespaceConventions=off
  Zero-Order Hold : ZeroOrderHold  SampleTime=publish_rate
  wires:
  Bus Assignment/1 -> Zero-Order Hold/1
  Blank Message/1 -> Bus Assignment/1
  Zero-Order Hold/1 -> Publish/1
  Demux/1 -> Bus Assignment/2
  Demux/2 -> Bus Assignment/3
  Demux/3 -> Bus Assignment/4
  p/1 -> Demux/1

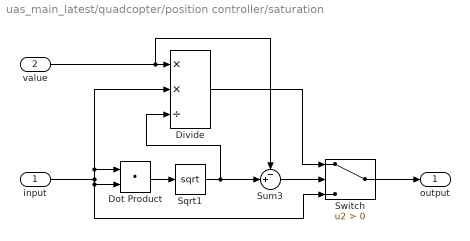
== system uas_main_latest/quadcopter/position controller/saturation ==
  input : Inport
  value : Inport  Port=2
  Divide : Product  Inputs=**/
  Dot Product : DotProduct  OutDataTypeStr=Inherit: Inherit via internal rule
  Sqrt1 : Sqrt
  Sum3 : Sum  Inputs=-+|
  Switch : Switch  Criteria=u2 > Threshold  SaturateOnIntegerOverflow=off  InputSameDT=off
  output : Outport
  wires:
  Divide/1 -> Switch/1
  value/1 -> Divide/1, Sum3/1
  Dot Product/1 -> Sqrt1/1
  Switch/1 -> output/1
  Sum3/1 -> Switch/2
  input/1 -> Switch/3, Dot Product/2, Divide/2, Dot Product/1
  Sqrt1/1 -> Sum3/2, Divide/3

== matlab function uas_main_latest/quadcopter/Attitude Controller/MATLAB Function1 ==
  data: roll input size=1; pitch input size=1; yaw input size=1; er output size=[3 1]; R input size=[3 3]
function er = lee(roll, pitch, yaw, R)

Rd = eul2rotm([yaw pitch roll], 'ZYX');

P = 1/2 * (Rd.' * R - R.' * Rd) ;

er = [P(3,2) ; P(1,3) ; P(2,1)] ;

== matlab function uas_main_latest/quadcopter/quat 2 euler (UE) ==
  data: q input size=[1 4]; attitude output
function attitude = euler_ue(q)

attitude = quat2eul(q, 'ZYX');

attitude = [attitude(1) attitude(2) attitude(3)];

== matlab function uas_main_latest/quadcopter/position controller/compute_roll_pitch ==
  data: F_d input; roll output; yaw_d input; pitch output
function [roll, pitch] = compute_roll_pitch(F_d, yaw_d)

yaw_dt = yaw_d + pi/2;
uyt = [cos(yaw_dt); sin(yaw_dt); 0];
uz = F_d/norm(F_d);
ux = cross(uyt, uz);
uy = cross(uz, ux);

attitude = rotm2eul([ux uy uz], 'ZYX');

roll = attitude(3);
pitch = attitude(2);

== stateflow chart uas_main_latest/waypoint navigation (Ex. 6.1 and 7.1) ==
  state go
    pd = [r(i, 1) ; r(i, 2) ; r(i, 3)]
  (default) -> go : {i = 1}
  go -> (junction 26) : [reached(pd, p)]
  (junction 26) -> go : [i < size(r, 1)]{i = i + 1}
  data: setpoint_position function_input; position function_input; is_reached function_output; r input; i local; p input; pd output size=[3 1]
  function is_reached = reached(setpoint_position, position):
    | function is_reached = reached(setpoint_position, position)
    | is_reached = norm(position - setpoint_position) < 0.1;

== matlab function uas_main_latest/quadcopter/quat 2 euler (ROS) ==
  data: q input size=[1 4]; roll_rad output; pitch_rad output; yaw_rad output
function [roll_rad, pitch_rad, yaw_rad] = euler_ros(q)

attitude = quat2eul(q, 'ZYX');

roll_rad = attitude(3);
pitch_rad = attitude(2);
yaw_rad = attitude(1);

== matlab function uas_main_latest/quadcopter/MATLAB Function ==
  data: u input; y output
function y = get33(u)

y = u(3,3);
